simulink model "watertank"  (Simulink 6.5)
settings: Solver=FixedStepDiscrete  StartTime=0.0  StopTime=200.0  FixedStep=0.1  RelTol=1e-3
PreLoadFcn:
  | watertankdat
settings Model: Creator=lparsons  LastModifiedBy=haf  ProdHWDeviceType=Specified
settings DataIOCC: SignalLoggingName=logsOut
settings OptimizationCC: InlineInvariantSignals=on
settings DebuggingCC: SolverPrmCheckMsg=none  MultiTaskDSMMsg=warning  StrictBusMsg=None
settings HardwareCC: ProdHWDeviceType=Specified

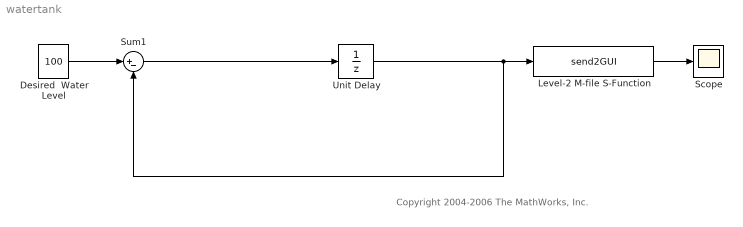
== system watertank ==
  note: Copyright 2004-2006 The MathWorks, Inc.
  Desired  Water Level : Constant  Value=100  OutDataType=sfix(16)  ConRadixGroup=Use specified scaling  OutScaling=2^0  SampleTime=inf  FramePeriod=inf
  Level-2 M-file S-Function : M-S-Function  FunctionName=send2GUI
  Scope : Scope
      settings: YMin=0  YMax=130
  Sum1 : Sum  Inputs=|+-  SaturateOnIntegerOverflow=on
  Unit Delay : UnitDelay
  wires:
  Desired  Water Level/1 -> Sum1/1
  Sum1/1 -> Unit Delay/1
  Unit Delay/1 -> Sum1/2, Level-2 M-file S-Function/1
  Level-2 M-file S-Function/1 -> Scope/1
